simulink model "SDV_HIL"  (R2025a)
settings: Solver=VariableStepAuto  StartTime=0.0  StopTime=9999  FixedStep=0.001  RelTol=1e-3
undefined symbols (not defined in the file): Breakpoints_Fz, Cij, dspblkCoreblockFVToolHelper, eta, Fx_total_max, g, gcbh, Iz, lambda, lf, lr, mu, phi, R_eff, Tmax, xi
libraries: simulink_extras x30, slrealtimeiplib x17, slpidlib x16, simulink x10, SignalEditorBlockLib x6, dspstat3 x5, Solver_SF x3, sl3dlib x3
(part 3 of 5)

== system SDV_HIL/Draft1/Subsystem1/Motor1/Subsystem ==
  In1 : Inport
  Add : Sum
  PID Controller : slpidlib/PID Controller  Controller=PID  Form=Parallel  TimeDomain=Continuous-time  UseExternalTs=off  SampleTime=0.001  IntegratorMethod=Forward Euler  FilterMethod=Forward Euler  ControllerParametersSource=internal  P=0  I=3.5024667128  UseKiTs=off  D=0  UseExternalDerivativeSource=off  N=100  UseFilter=on  TunerSelectOption=Transfer Function Based (PID Tuner App)  InitialConditionSource=internal  InitialConditionForIntegrator=0  InitialConditionForFilter=0  DifferentiatorICPrevScaledInput=0  ExternalReset=none  TrackingMode=off  Kt=1  LimitOutput=off  SatLimitsSource=internal  UpperSaturationLimit=inf  LowerSaturationLimit=-inf  LinearizeAsGain=on  AntiWindupMode=none  Kb=1  LimitIntegrator=off  UpperIntegratorSaturationLimit=inf  LowerIntegratorSaturationLimit=-inf  POutMin=[]  POutMax=[]  IOutMin=[]  IOutMax=[]  DOutMin=[]  DOutMax=[]  NOutMin=[]  NOutMax=[]  SumOutMin=[]  SumOutMax=[]  SaturationOutMin=[]  SaturationOutMax=[]  PParamMin=[]  PParamMax=[]  IParamMin=[]  IParamMax=[]  DParamMin=[]  DParamMax=[]  NParamMin=[]  NParamMax=[]  KbParamMin=[]  KbParamMax=[]  KtParamMin=[]  KtParamMax=[]  KbOutMin=[]  KbOutMax=[]  KtOutMin=[]  KtOutMax=[]  IntegratorOutMin=[]  IntegratorOutMax=[]  FilterOutMin=[]  FilterOutMax=[]  SumI1OutMin=[]  SumI1OutMax=[]  SumI2OutMin=[]  SumI2OutMax=[]  SumI3OutMin=[]  SumI3OutMax=[]  SumI4OutMin=[]  SumI4OutMax=[]  SumDOutMin=[]  SumDOutMax=[]  DifferentiatorOutMin=[]  DifferentiatorOutMax=[]  FilterDiffOutCoefMin=[]  FilterDiffOutCoefMax=[]  ReciprocalOutMin=[]  ReciprocalOutMax=[]  SumDenOutMin=[]  SumDenOutMax=[]  SumNumOutMin=[]  SumNumOutMax=[]  DivideOutMin=[]  DivideOutMax=[]  UdiffTsProdOutMin=[]  UdiffTsProdOutMax=[]  NTsProdOutMin=[]  NTsProdOutMax=[]  UintegralTsProdOutMin=[]  UintegralTsProdOutMax=[]  UngainTsProdOutMin=[]  UngainTsProdOutMax=[]  ClampingZeroOutDataTypeStr=Inherit: Inherit via back propagation  ClampingZeroOutMin=[]  ClampingZeroOutMax=[]  FilterDenConstantOutDataTypeStr=Inherit: Inherit via back propagation  FilterDenConstantOutMin=[]  FilterDenConstantOutMax=[]  PCopyOutDataTypeStr=Inherit: Inherit via back propagation  PCopyOutMin=[]  PCopyOutMax=[]  NCopyOutDataTypeStr=Inherit: Inherit via back propagation  NCopyOutMin=[]  NCopyOutMax=[]  IntegratorContinuousStateAttributes=''  IntegratorStateMustResolveToSignalObject=off  IntegratorRTWStateStorageClass=Auto  FilterContinuousStateAttributes=''  FilterStateMustResolveToSignalObject=off  FilterRTWStateStorageClass=Auto  ParallelPVariant=InternalParameters  IdealPVariant=Disabled  IVariant=InternalParameters  DVariant=InternalParameters  IntegratorVariant=Continuous  SatVariant=Disabled  AWVariant=Passthrough  PCopyVariant=Disabled  TRVariant=Disabled  FdbkBlocksVariant=Forward  IdealPFdbkVariant=Disabled  SatFdbkVariant=Disabled  DerivativeFilterVariant=ContFilter  NVariant=InternalParameters  NCopyVariant=Disabled  FilterICVariant=InternalICsFilter  IntegratorICVariant=InternalICs  ExternalResetVariant=Disabled  TRSumVariant=Passthrough  SumFdbkVariant=Disabled  SumVariant=Sum_PID  TsampFilterVariant=InternalTs  TsampNgainVariant=Passthrough  TsampIntegralVariant=Disabled_SignalSpec  ExternalSaturationOutDataTypeStr=Inherit: Same as second input  DerivativeSourceVariant=ErrorSignal  PreIntVariant=InternalPreInt
  Saturation : Saturate  UpperLimit=110  LowerLimit=-110
  Scope : Scope
      settings: ActiveDisplayYMinimum=-13.749999999999996  ActiveDisplayYMaximum=123.75  DataLoggingVariableName=ScopeData10
  Scope1 : Scope  NumInputPorts=2
      settings: ActiveDisplayYMinimum=-21.066394763656298  ActiveDisplayYMaximum=122.34078579666662  DataLoggingVariableName=ScopeData13
  Scope2 : Scope
      settings: ActiveDisplayYMinimum=-17.082157059379561  ActiveDisplayYMaximum=107.74564424656792  DataLoggingVariableName=ScopeData16
  Sum : Sum  Inputs=|+-
  Temporary DC Motor model3 : TransferFcn  Numerator=[-146.29,3022.7]  Denominator=[1,117.06,3078.7]
  Out1 : Outport
  wires:
  [initialCondition] -> Add/2
  Add/1 -> Out1/1, Sum/2, Scope1/2, Scope2/1
  Temporary DC Motor model3/1 -> Add/1
  Saturation/1 -> Temporary DC Motor model3/1, Scope/1
  In1/1 -> Sum/1, Scope1/1
  Sum/1 -> PID Controller/1
  PID Controller/1 -> Saturation/1

== system SDV_HIL/Draft1/Subsystem1/Motor1/Subsystem1 ==
  In1 : Inport
  Add : Sum
  PID Controller : slpidlib/PID Controller  Controller=PID  Form=Parallel  TimeDomain=Continuous-time  UseExternalTs=off  SampleTime=0.001  IntegratorMethod=Forward Euler  FilterMethod=Forward Euler  ControllerParametersSource=internal  P=0  I=3.5024667128  UseKiTs=off  D=0  UseExternalDerivativeSource=off  N=100  UseFilter=on  TunerSelectOption=Transfer Function Based (PID Tuner App)  InitialConditionSource=internal  InitialConditionForIntegrator=0  InitialConditionForFilter=0  DifferentiatorICPrevScaledInput=0  ExternalReset=none  TrackingMode=off  Kt=1  LimitOutput=off  SatLimitsSource=internal  UpperSaturationLimit=inf  LowerSaturationLimit=-inf  LinearizeAsGain=on  AntiWindupMode=none  Kb=1  LimitIntegrator=off  UpperIntegratorSaturationLimit=inf  LowerIntegratorSaturationLimit=-inf  POutMin=[]  POutMax=[]  IOutMin=[]  IOutMax=[]  DOutMin=[]  DOutMax=[]  NOutMin=[]  NOutMax=[]  SumOutMin=[]  SumOutMax=[]  SaturationOutMin=[]  SaturationOutMax=[]  PParamMin=[]  PParamMax=[]  IParamMin=[]  IParamMax=[]  DParamMin=[]  DParamMax=[]  NParamMin=[]  NParamMax=[]  KbParamMin=[]  KbParamMax=[]  KtParamMin=[]  KtParamMax=[]  KbOutMin=[]  KbOutMax=[]  KtOutMin=[]  KtOutMax=[]  IntegratorOutMin=[]  IntegratorOutMax=[]  FilterOutMin=[]  FilterOutMax=[]  SumI1OutMin=[]  SumI1OutMax=[]  SumI2OutMin=[]  SumI2OutMax=[]  SumI3OutMin=[]  SumI3OutMax=[]  SumI4OutMin=[]  SumI4OutMax=[]  SumDOutMin=[]  SumDOutMax=[]  DifferentiatorOutMin=[]  DifferentiatorOutMax=[]  FilterDiffOutCoefMin=[]  FilterDiffOutCoefMax=[]  ReciprocalOutMin=[]  ReciprocalOutMax=[]  SumDenOutMin=[]  SumDenOutMax=[]  SumNumOutMin=[]  SumNumOutMax=[]  DivideOutMin=[]  DivideOutMax=[]  UdiffTsProdOutMin=[]  UdiffTsProdOutMax=[]  NTsProdOutMin=[]  NTsProdOutMax=[]  UintegralTsProdOutMin=[]  UintegralTsProdOutMax=[]  UngainTsProdOutMin=[]  UngainTsProdOutMax=[]  ClampingZeroOutDataTypeStr=Inherit: Inherit via back propagation  ClampingZeroOutMin=[]  ClampingZeroOutMax=[]  FilterDenConstantOutDataTypeStr=Inherit: Inherit via back propagation  FilterDenConstantOutMin=[]  FilterDenConstantOutMax=[]  PCopyOutDataTypeStr=Inherit: Inherit via back propagation  PCopyOutMin=[]  PCopyOutMax=[]  NCopyOutDataTypeStr=Inherit: Inherit via back propagation  NCopyOutMin=[]  NCopyOutMax=[]  IntegratorContinuousStateAttributes=''  IntegratorStateMustResolveToSignalObject=off  IntegratorRTWStateStorageClass=Auto  FilterContinuousStateAttributes=''  FilterStateMustResolveToSignalObject=off  FilterRTWStateStorageClass=Auto  ParallelPVariant=InternalParameters  IdealPVariant=Disabled  IVariant=InternalParameters  DVariant=InternalParameters  IntegratorVariant=Continuous  SatVariant=Disabled  AWVariant=Passthrough  PCopyVariant=Disabled  TRVariant=Disabled  FdbkBlocksVariant=Forward  IdealPFdbkVariant=Disabled  SatFdbkVariant=Disabled  DerivativeFilterVariant=ContFilter  NVariant=InternalParameters  NCopyVariant=Disabled  FilterICVariant=InternalICsFilter  IntegratorICVariant=InternalICs  ExternalResetVariant=Disabled  TRSumVariant=Passthrough  SumFdbkVariant=Disabled  SumVariant=Sum_PID  TsampFilterVariant=InternalTs  TsampNgainVariant=Passthrough  TsampIntegralVariant=Disabled_SignalSpec  ExternalSaturationOutDataTypeStr=Inherit: Same as second input  DerivativeSourceVariant=ErrorSignal  PreIntVariant=InternalPreInt
  Saturation : Saturate  UpperLimit=110  LowerLimit=-110
  Scope : Scope
      settings: ActiveDisplayYMinimum=-1  ActiveDisplayYMaximum=1  DataLoggingVariableName=ScopeData10
  Scope1 : Scope  NumInputPorts=2
      settings: ActiveDisplayYMinimum=70.760540850772571  ActiveDisplayYMaximum=162.62283553098897  DataLoggingVariableName=ScopeData13
  Scope2 : Scope
      settings: ActiveDisplayYMinimum=-1  ActiveDisplayYMaximum=1  DataLoggingVariableName=ScopeData16
  Sum : Sum  Inputs=|+-
  Temporary DC Motor model3 : TransferFcn  Numerator=[-146.29,3022.7]  Denominator=[1,117.06,3078.7]
  Out1 : Outport
  wires:
  PID Controller/1 -> Saturation/1
  Sum/1 -> PID Controller/1
  In1/1 -> Scope1/1, Sum/1
  Saturation/1 -> Scope/1, Temporary DC Motor model3/1
  Temporary DC Motor model3/1 -> Add/1
  Add/1 -> Scope2/1, Scope1/2, Sum/2, Out1/1
  [initialCondition] -> Add/2

== system SDV_HIL/Draft1/Subsystem1/Motor1/Subsystem2 ==
  In1 : Inport
  Add : Sum
  PID Controller : slpidlib/PID Controller  Controller=PID  Form=Parallel  TimeDomain=Continuous-time  UseExternalTs=off  SampleTime=0.001  IntegratorMethod=Forward Euler  FilterMethod=Forward Euler  ControllerParametersSource=internal  P=0  I=3.5024667128  UseKiTs=off  D=0  UseExternalDerivativeSource=off  N=100  UseFilter=on  TunerSelectOption=Transfer Function Based (PID Tuner App)  InitialConditionSource=internal  InitialConditionForIntegrator=0  InitialConditionForFilter=0  DifferentiatorICPrevScaledInput=0  ExternalReset=none  TrackingMode=off  Kt=1  LimitOutput=off  SatLimitsSource=internal  UpperSaturationLimit=inf  LowerSaturationLimit=-inf  LinearizeAsGain=on  AntiWindupMode=none  Kb=1  LimitIntegrator=off  UpperIntegratorSaturationLimit=inf  LowerIntegratorSaturationLimit=-inf  POutMin=[]  POutMax=[]  IOutMin=[]  IOutMax=[]  DOutMin=[]  DOutMax=[]  NOutMin=[]  NOutMax=[]  SumOutMin=[]  SumOutMax=[]  SaturationOutMin=[]  SaturationOutMax=[]  PParamMin=[]  PParamMax=[]  IParamMin=[]  IParamMax=[]  DParamMin=[]  DParamMax=[]  NParamMin=[]  NParamMax=[]  KbParamMin=[]  KbParamMax=[]  KtParamMin=[]  KtParamMax=[]  KbOutMin=[]  KbOutMax=[]  KtOutMin=[]  KtOutMax=[]  IntegratorOutMin=[]  IntegratorOutMax=[]  FilterOutMin=[]  FilterOutMax=[]  SumI1OutMin=[]  SumI1OutMax=[]  SumI2OutMin=[]  SumI2OutMax=[]  SumI3OutMin=[]  SumI3OutMax=[]  SumI4OutMin=[]  SumI4OutMax=[]  SumDOutMin=[]  SumDOutMax=[]  DifferentiatorOutMin=[]  DifferentiatorOutMax=[]  FilterDiffOutCoefMin=[]  FilterDiffOutCoefMax=[]  ReciprocalOutMin=[]  ReciprocalOutMax=[]  SumDenOutMin=[]  SumDenOutMax=[]  SumNumOutMin=[]  SumNumOutMax=[]  DivideOutMin=[]  DivideOutMax=[]  UdiffTsProdOutMin=[]  UdiffTsProdOutMax=[]  NTsProdOutMin=[]  NTsProdOutMax=[]  UintegralTsProdOutMin=[]  UintegralTsProdOutMax=[]  UngainTsProdOutMin=[]  UngainTsProdOutMax=[]  ClampingZeroOutDataTypeStr=Inherit: Inherit via back propagation  ClampingZeroOutMin=[]  ClampingZeroOutMax=[]  FilterDenConstantOutDataTypeStr=Inherit: Inherit via back propagation  FilterDenConstantOutMin=[]  FilterDenConstantOutMax=[]  PCopyOutDataTypeStr=Inherit: Inherit via back propagation  PCopyOutMin=[]  PCopyOutMax=[]  NCopyOutDataTypeStr=Inherit: Inherit via back propagation  NCopyOutMin=[]  NCopyOutMax=[]  IntegratorContinuousStateAttributes=''  IntegratorStateMustResolveToSignalObject=off  IntegratorRTWStateStorageClass=Auto  FilterContinuousStateAttributes=''  FilterStateMustResolveToSignalObject=off  FilterRTWStateStorageClass=Auto  ParallelPVariant=InternalParameters  IdealPVariant=Disabled  IVariant=InternalParameters  DVariant=InternalParameters  IntegratorVariant=Continuous  SatVariant=Disabled  AWVariant=Passthrough  PCopyVariant=Disabled  TRVariant=Disabled  FdbkBlocksVariant=Forward  IdealPFdbkVariant=Disabled  SatFdbkVariant=Disabled  DerivativeFilterVariant=ContFilter  NVariant=InternalParameters  NCopyVariant=Disabled  FilterICVariant=InternalICsFilter  IntegratorICVariant=InternalICs  ExternalResetVariant=Disabled  TRSumVariant=Passthrough  SumFdbkVariant=Disabled  SumVariant=Sum_PID  TsampFilterVariant=InternalTs  TsampNgainVariant=Passthrough  TsampIntegralVariant=Disabled_SignalSpec  ExternalSaturationOutDataTypeStr=Inherit: Same as second input  DerivativeSourceVariant=ErrorSignal  PreIntVariant=InternalPreInt
  Saturation : Saturate  UpperLimit=110  LowerLimit=-110
  Scope : Scope
      settings: ActiveDisplayYMinimum=-1  ActiveDisplayYMaximum=1  DataLoggingVariableName=ScopeData10
  Scope1 : Scope  NumInputPorts=2
      settings: ActiveDisplayYMinimum=70.760540850772571  ActiveDisplayYMaximum=162.62283553098897  DataLoggingVariableName=ScopeData13
  Scope2 : Scope
      settings: ActiveDisplayYMinimum=-1  ActiveDisplayYMaximum=1  DataLoggingVariableName=ScopeData16
  Sum : Sum  Inputs=|+-
  Temporary DC Motor model3 : TransferFcn  Numerator=[-146.29,3022.7]  Denominator=[1,117.06,3078.7]
  Out1 : Outport
  wires:
  [initialCondition] -> Add/2
  Add/1 -> Out1/1, Sum/2, Scope1/2, Scope2/1
  Temporary DC Motor model3/1 -> Add/1
  Saturation/1 -> Temporary DC Motor model3/1, Scope/1
  In1/1 -> Sum/1, Scope1/1
  Sum/1 -> PID Controller/1
  PID Controller/1 -> Saturation/1

== system SDV_HIL/Draft1/Subsystem1/Motor1/Subsystem3 ==
  In1 : Inport
  Add : Sum
  PID Controller : slpidlib/PID Controller  Controller=PID  Form=Parallel  TimeDomain=Continuous-time  UseExternalTs=off  SampleTime=0.001  IntegratorMethod=Forward Euler  FilterMethod=Forward Euler  ControllerParametersSource=internal  P=0  I=3.5024667128  UseKiTs=off  D=0  UseExternalDerivativeSource=off  N=100  UseFilter=on  TunerSelectOption=Transfer Function Based (PID Tuner App)  InitialConditionSource=internal  InitialConditionForIntegrator=0  InitialConditionForFilter=0  DifferentiatorICPrevScaledInput=0  ExternalReset=none  TrackingMode=off  Kt=1  LimitOutput=off  SatLimitsSource=internal  UpperSaturationLimit=inf  LowerSaturationLimit=-inf  LinearizeAsGain=on  AntiWindupMode=none  Kb=1  LimitIntegrator=off  UpperIntegratorSaturationLimit=inf  LowerIntegratorSaturationLimit=-inf  POutMin=[]  POutMax=[]  IOutMin=[]  IOutMax=[]  DOutMin=[]  DOutMax=[]  NOutMin=[]  NOutMax=[]  SumOutMin=[]  SumOutMax=[]  SaturationOutMin=[]  SaturationOutMax=[]  PParamMin=[]  PParamMax=[]  IParamMin=[]  IParamMax=[]  DParamMin=[]  DParamMax=[]  NParamMin=[]  NParamMax=[]  KbParamMin=[]  KbParamMax=[]  KtParamMin=[]  KtParamMax=[]  KbOutMin=[]  KbOutMax=[]  KtOutMin=[]  KtOutMax=[]  IntegratorOutMin=[]  IntegratorOutMax=[]  FilterOutMin=[]  FilterOutMax=[]  SumI1OutMin=[]  SumI1OutMax=[]  SumI2OutMin=[]  SumI2OutMax=[]  SumI3OutMin=[]  SumI3OutMax=[]  SumI4OutMin=[]  SumI4OutMax=[]  SumDOutMin=[]  SumDOutMax=[]  DifferentiatorOutMin=[]  DifferentiatorOutMax=[]  FilterDiffOutCoefMin=[]  FilterDiffOutCoefMax=[]  ReciprocalOutMin=[]  ReciprocalOutMax=[]  SumDenOutMin=[]  SumDenOutMax=[]  SumNumOutMin=[]  SumNumOutMax=[]  DivideOutMin=[]  DivideOutMax=[]  UdiffTsProdOutMin=[]  UdiffTsProdOutMax=[]  NTsProdOutMin=[]  NTsProdOutMax=[]  UintegralTsProdOutMin=[]  UintegralTsProdOutMax=[]  UngainTsProdOutMin=[]  UngainTsProdOutMax=[]  ClampingZeroOutDataTypeStr=Inherit: Inherit via back propagation  ClampingZeroOutMin=[]  ClampingZeroOutMax=[]  FilterDenConstantOutDataTypeStr=Inherit: Inherit via back propagation  FilterDenConstantOutMin=[]  FilterDenConstantOutMax=[]  PCopyOutDataTypeStr=Inherit: Inherit via back propagation  PCopyOutMin=[]  PCopyOutMax=[]  NCopyOutDataTypeStr=Inherit: Inherit via back propagation  NCopyOutMin=[]  NCopyOutMax=[]  IntegratorContinuousStateAttributes=''  IntegratorStateMustResolveToSignalObject=off  IntegratorRTWStateStorageClass=Auto  FilterContinuousStateAttributes=''  FilterStateMustResolveToSignalObject=off  FilterRTWStateStorageClass=Auto  ParallelPVariant=InternalParameters  IdealPVariant=Disabled  IVariant=InternalParameters  DVariant=InternalParameters  IntegratorVariant=Continuous  SatVariant=Disabled  AWVariant=Passthrough  PCopyVariant=Disabled  TRVariant=Disabled  FdbkBlocksVariant=Forward  IdealPFdbkVariant=Disabled  SatFdbkVariant=Disabled  DerivativeFilterVariant=ContFilter  NVariant=InternalParameters  NCopyVariant=Disabled  FilterICVariant=InternalICsFilter  IntegratorICVariant=InternalICs  ExternalResetVariant=Disabled  TRSumVariant=Passthrough  SumFdbkVariant=Disabled  SumVariant=Sum_PID  TsampFilterVariant=InternalTs  TsampNgainVariant=Passthrough  TsampIntegralVariant=Disabled_SignalSpec  ExternalSaturationOutDataTypeStr=Inherit: Same as second input  DerivativeSourceVariant=ErrorSignal  PreIntVariant=InternalPreInt
  Saturation : Saturate  UpperLimit=110  LowerLimit=-110
  Scope : Scope
      settings: ActiveDisplayYMinimum=-1  ActiveDisplayYMaximum=1  DataLoggingVariableName=ScopeData10
  Scope1 : Scope  NumInputPorts=2
      settings: ActiveDisplayYMinimum=70.760540850772571  ActiveDisplayYMaximum=162.62283553098897  DataLoggingVariableName=ScopeData13
  Scope2 : Scope
      settings: ActiveDisplayYMinimum=-1  ActiveDisplayYMaximum=1  DataLoggingVariableName=ScopeData16
  Sum : Sum  Inputs=|+-
  Temporary DC Motor model3 : TransferFcn  Numerator=[-146.29,3022.7]  Denominator=[1,117.06,3078.7]
  Out1 : Outport
  wires:
  PID Controller/1 -> Saturation/1
  Sum/1 -> PID Controller/1
  In1/1 -> Scope1/1, Sum/1
  Saturation/1 -> Scope/1, Temporary DC Motor model3/1
  Temporary DC Motor model3/1 -> Add/1
  Add/1 -> Scope2/1, Scope1/2, Sum/2, Out1/1
  [initialCondition] -> Add/2

== system SDV_HIL/Draft1/Subsystem1/Motor1/Traction Control ==
  SpdTCS : Inport
  Add : Sum
  Add1 : Sum
  Mux : Mux  Inputs=2
  Scope1 : Scope
      settings: ActiveDisplayYMinimum=-42.212003619613114  ActiveDisplayYMaximum=156.59295699794211  DataLoggingVariableName=ScopeData29
  Selector : Selector  InputPortWidth=4  IndexOptions=Index vector (dialog)  Indices=[1 2]  OutputSizes=1
  Selector1 : Selector  InputPortWidth=4  IndexOptions=Index vector (dialog)  Indices=[3 4]  OutputSizes=1
  Slip Calculation : Subsystem
  Slip Calculation1 : Subsystem
  Subsystem : Subsystem
  Subsystem1 : Subsystem
  Out1 : Outport
  wires:
  Subsystem1/1(y) -> Add1/2
  Slip Calculation1/1(slip) -> Subsystem1/1(slip)
  Slip Calculation/1(slip) -> Subsystem/1(In1)
  Subsystem/1(y) -> Add/2
  Add/1 -> Mux/1
  Add1/1 -> Mux/2
  Mux/1 -> Out1/1, Scope1/1
  Selector1/1 -> Add1/1
  Selector/1 -> Add/1
  SpdTCS/1 -> Selector1/1, Selector/1

== system SDV_HIL/Draft1/Subsystem1/Steering1/Cr, calculation ==
  In1 : Inport
  Add : Sum
  Add1 : Sum
  Demux : Demux  Outputs=2
  Divide : Product  Inputs=*/
  Divide1 : Product  Inputs=*/
  Divide2 : Product  Inputs=*/
  Scope1 : Scope
      settings: ActiveDisplayYMinimum=-33.245119024843021  ActiveDisplayYMaximum=11.158574802269591  DataLoggingVariableName=ScopeData36
  Scope2 : Scope  NumInputPorts=3
      settings: ActiveDisplayYMinimum=-11896.025438814215  ActiveDisplayYMaximum=9098.0677384906721  DataLoggingVariableName=ScopeData37
  Scope3 : Scope  NumInputPorts=2
      settings: ActiveDisplayYMinimum=-1372.0128718321157  ActiveDisplayYMaximum=6027.9532460136825  DataLoggingVariableName=ScopeData39
  Scope4 : Scope
      settings: ActiveDisplayYMinimum=-1233.3601043062406  ActiveDisplayYMaximum=4986.210757668915  DataLoggingVariableName=ScopeData46
  Scope5 : Scope
      settings: ActiveDisplayYMinimum=-54160.327682168427  ActiveDisplayYMaximum=53171.641125613256  DataLoggingVariableName=ScopeData12
  Selector : Selector  InputPortWidth=4  IndexOptions=Index vector (dialog)  Indices=[3 4]  OutputSizes=1
  Subsystem : Subsystem
  wires:
  Add1/1 -> Scope5/1  "Cr"
  [sideslip_R2] -> Divide2/2
  Divide2/1 -> Add1/2  "Cr_R2"
  Divide1/1 -> Add1/1  "Cr_L2"
  [sideslip_L2] -> Divide1/2
  Divide/1 -> Scope2/2  "Cr"
  Add/1 -> Divide/1, Scope2/1, Scope3/2
  Selector/1 -> Demux/1, Scope3/1
  Demux/2 -> Add/2, Divide2/1
  Subsystem/1(Out1) -> Scope1/1, Scope2/3, Divide/2  "ar, side slip rear"
  [Fy] -> Selector/1, Scope4/1
  Demux/1 -> Divide1/1, Add/1
  In1/1 -> Subsystem/1(In1)

== system SDV_HIL/Draft1/Subsystem1/Steering1/Dynamic ==
  In2 : Inport
  Mz : Inport  Port=2
  Demux : Demux
  Mux : Mux
  PID Controller{,1..3} (4 alike) : slpidlib/PID Controller  Controller=PD  Form=Parallel  TimeDomain=Continuous-time  UseExternalTs=off  SampleTime=-1  IntegratorMethod=Forward Euler  FilterMethod=Forward Euler  ControllerParametersSource=internal  P=447.054647999311  I=1.94153008706553  UseKiTs=off  D=0  UseExternalDerivativeSource=off  N=100  UseFilter=on  TunerSelectOption=Transfer Function Based (PID Tuner App)  InitialConditionSource=internal  InitialConditionForIntegrator=0  InitialConditionForFilter=0  DifferentiatorICPrevScaledInput=0  ExternalReset=none  TrackingMode=off  Kt=1  LimitOutput=off  SatLimitsSource=internal  UpperSaturationLimit=inf  LowerSaturationLimit=-inf  LinearizeAsGain=on  AntiWindupMode=none  Kb=1  LimitIntegrator=off  UpperIntegratorSaturationLimit=inf  LowerIntegratorSaturationLimit=-inf  POutMin=[]  POutMax=[]  IOutMin=[]  IOutMax=[]  DOutMin=[]  DOutMax=[]  NOutMin=[]  NOutMax=[]  SumOutMin=[]  SumOutMax=[]  SaturationOutMin=[]  SaturationOutMax=[]  PParamMin=[]  PParamMax=[]  IParamMin=[]  IParamMax=[]  DParamMin=[]  DParamMax=[]  NParamMin=[]  NParamMax=[]  KbParamMin=[]  KbParamMax=[]  KtParamMin=[]  KtParamMax=[]  KbOutMin=[]  KbOutMax=[]  KtOutMin=[]  KtOutMax=[]  IntegratorOutMin=[]  IntegratorOutMax=[]  FilterOutMin=[]  FilterOutMax=[]  SumI1OutMin=[]  SumI1OutMax=[]  SumI2OutMin=[]  SumI2OutMax=[]  SumI3OutMin=[]  SumI3OutMax=[]  SumI4OutMin=[]  SumI4OutMax=[]  SumDOutMin=[]  SumDOutMax=[]  DifferentiatorOutMin=[]  DifferentiatorOutMax=[]  FilterDiffOutCoefMin=[]  FilterDiffOutCoefMax=[]  ReciprocalOutMin=[]  ReciprocalOutMax=[]  SumDenOutMin=[]  SumDenOutMax=[]  SumNumOutMin=[]  SumNumOutMax=[]  DivideOutMin=[]  DivideOutMax=[]  UdiffTsProdOutMin=[]  UdiffTsProdOutMax=[]  NTsProdOutMin=[]  NTsProdOutMax=[]  UintegralTsProdOutMin=[]  UintegralTsProdOutMax=[]  UngainTsProdOutMin=[]  UngainTsProdOutMax=[]  ClampingZeroOutDataTypeStr=Inherit: Inherit via back propagation  ClampingZeroOutMin=[]  ClampingZeroOutMax=[]  FilterDenConstantOutDataTypeStr=Inherit: Inherit via back propagation  FilterDenConstantOutMin=[]  FilterDenConstantOutMax=[]  PCopyOutDataTypeStr=Inherit: Inherit via back propagation  PCopyOutMin=[]  PCopyOutMax=[]  NCopyOutDataTypeStr=Inherit: Inherit via back propagation  NCopyOutMin=[]  NCopyOutMax=[]  IntegratorContinuousStateAttributes=''  IntegratorStateMustResolveToSignalObject=off  IntegratorRTWStateStorageClass=Auto  FilterContinuousStateAttributes=''  FilterStateMustResolveToSignalObject=off  FilterRTWStateStorageClass=Auto  ParallelPVariant=InternalParameters  IdealPVariant=Disabled  IVariant=Disabled  DVariant=InternalParameters  IntegratorVariant=Disabled  SatVariant=Disabled  AWVariant=Disabled  PCopyVariant=Disabled  TRVariant=Disabled  FdbkBlocksVariant=Forward  IdealPFdbkVariant=Disabled  SatFdbkVariant=Disabled  DerivativeFilterVariant=ContFilter  NVariant=InternalParameters  NCopyVariant=Disabled  FilterICVariant=InternalICsFilter  IntegratorICVariant=Disabled  ExternalResetVariant=Disabled  TRSumVariant=Passthrough  SumFdbkVariant=Disabled  SumVariant=Sum_PD  TsampFilterVariant=InternalTs  TsampNgainVariant=Passthrough  TsampIntegralVariant=Disabled_SignalSpec  ExternalSaturationOutDataTypeStr=Inherit: Same as second input  DerivativeSourceVariant=ErrorSignal  PreIntVariant=InternalPreInt
  Scope{,1..3} (4 alike) : Scope  NumInputPorts=2
      Scope settings: ActiveDisplayYMinimum=-1  ActiveDisplayYMaximum=1
      Scope1 settings: ActiveDisplayYMinimum=1.8720993876921048  ActiveDisplayYMaximum=2.8130930610708664  DataLoggingVariableName=ScopeData32
      Scope2 settings: ActiveDisplayYMinimum=-18267.79992914902  ActiveDisplayYMaximum=55993.76279968489  DataLoggingVariableName=ScopeData58
      Scope3 settings: ActiveDisplayYMinimum=-0.014012303296182898  ActiveDisplayYMaximum=0.010807485381998104  DataLoggingVariableName=ScopeData59
  Steering cmd : Subsystem
  Sum{,1..5} (6 alike) : Sum  Inputs=|+-
  Temporary Stepper Motor model{1..4} (4 alike) : TransferFcn  Numerator=[80.823,1752.8]  Denominator=[1,177.23,1759.6]
  Deg : Outport
  wires:
  Sum2/1 -> Scope3/1, PID Controller2/1
  Sum3/1 -> PID Controller3/1, Scope3/2
  Steering cmd/1(Out1) -> Sum5/2, Sum4/2
  Sum5/1 -> Scope/2, Sum3/1
  Demux/4 -> Sum5/1
  Sum4/1 -> Scope/1, Sum2/1
  Demux/3 -> Sum4/1
  Mz/1 -> Steering cmd/1(In1)
  Demux/2 -> Sum1/1
  Sum1/1 -> PID Controller1/1
  Demux/1 -> Sum/1
  Sum/1 -> PID Controller/1
  PID Controller3/1 -> Temporary Stepper Motor model4/1, Scope2/2
  PID Controller2/1 -> Temporary Stepper Motor model3/1, Scope2/1
  PID Controller1/1 -> Temporary Stepper Motor model2/1
  PID Controller/1 -> Temporary Stepper Motor model1/1
  Mux/1 -> Deg/1
  Temporary Stepper Motor model4/1 -> Mux/4, Scope1/1, Sum3/2
  Temporary Stepper Motor model3/1 -> Mux/3, Scope1/2, Sum2/2
  Temporary Stepper Motor model2/1 -> Mux/2, Sum1/2
  Temporary Stepper Motor model1/1 -> Mux/1, Sum/2
  In2/1 -> Demux/1

== system SDV_HIL/Draft1/UDP Transmit PC -> VCU1/Subsystem/4 Wheel Steering system ==
  Spd : Inport
  Str : Inport  Port=2
  Display : Display
  Display1 : Display
  Kinematik : Subsystem
  Ang_reff : Outport
  wires:
  Kinematik/2(YO) -> Display/1
  Kinematik/3(XO) -> Display1/1
  Str/1 -> Kinematik/2(Steer)
  Spd/1 -> Kinematik/1(Speed)
  Kinematik/1(Out1) -> Ang_reff/1

== system SDV_HIL/Draft1/UDP Transmit PC -> VCU1/Subsystem/Torque Vectoring ==
  Vx_des : Inport
  Vx : Inport  Port=2
  Vy : Inport  Port=3
  AngWheel : Inport  Port=4
  r : Inport  Port=5
  Fy : Inport  Port=6
  Fz : Inport  Port=7  PortDimensions=[4 1]
  Ca Calculations : Subsystem
  Constant : Constant  Value=0
  Lower-Level Control : Subsystem
      settings: PortSchema="{\"entries\":[{\"content\":{\"sides\":[{\"content\":{\"connectorIds\":[\"In1\",\"In2\"]},\"type\":\"ConnectorPlacement.EquallySpacedRectSide\",\"uuid\":\"57e37133-a4ce-4bcd-b7d5-2c7ad964fba5\"},{\"content\":{\"connectorIds\":[\"Out1\"],\"side\":\"RIGHT\"},\"type\":\"ConnectorPlacement.EquallySpacedRectSide\",\"uuid\":\"b1a2d58e-03dd-4a8c-b0ff-f0fba1e94d60\"},{\"content\":{\"side\":\"TOP\"},\"type\":\"ConnectorPlacement.EquallySpacedRectSide\",\"uuid\":\"ceca0281-a87d-4fe2-92d9-19deb493506e\"},{\"content\":{\"connectorIds\":[\"In3\",\"In4\"],\"side\":\"BOTTOM\"},\"type\":\"ConnectorPlacement.EquallySpacedRectSide\",\"uuid\":\"a2fed640-7310-4b0a-b340-bd8e53025f92\"}]},\"type\":\"ConnectorPlacement.EquallySpacedConnector\",\"uuid\":\"a7bc2132-8edf-46cf-bd03-69d09e070427\"}],\"packageUris\":[\"http://schema.mathworks.com/mf0/Connector/R2020b\"],\"version\":\"1.0\"}"
  Reference Model : Subsystem
  Scope1 : Scope  Commented=on
      settings: TimeSpan=10  ActiveDisplayYMinimum=-27041.642916219451  ActiveDisplayYMaximum=46357.700395381871  DataLoggingVariableName=ScopeData5
  Scope2 : Scope  Commented=on
      settings: TimeSpan=10  ActiveDisplayYMinimum=-266.81339424220005  ActiveDisplayYMaximum=314.09270908605555  DataLoggingVariableName=ScopeData7
  Speed Control : Subsystem
  Terminator : Terminator
  Upper-Level Control : Subsystem
      settings: PortSchema="{\"entries\":[{\"content\":{\"sides\":[{\"content\":{\"connectorIds\":[\"In1\",\"In2\"]},\"type\":\"ConnectorPlacement.EquallySpacedRectSide\",\"uuid\":\"0439ec5c-b28f-4113-9d52-608e9559868e\"},{\"content\":{\"connectorIds\":[\"Out1\"],\"side\":\"RIGHT\"},\"type\":\"ConnectorPlacement.EquallySpacedRectSide\",\"uuid\":\"fb34909b-3fa5-4238-9bd9-6fa6bbc40fd8\"},{\"content\":{\"side\":\"TOP\"},\"type\":\"ConnectorPlacement.EquallySpacedRectSide\",\"uuid\":\"fd4c258c-89bb-45ab-b8b8-d01502b1a89c\"},{\"content\":{\"connectorIds\":[\"In3\",\"In4\",\"In5\",\"In6\"],\"side\":\"BOTTOM\"},\"type\":\"ConnectorPlacement.EquallySpacedRectSide\",\"uuid\":\"b800e5eb-1f42-45fc-807a-e4c0534ff65a\"}]},\"type\":\"ConnectorPlacement.EquallySpacedConnector\",\"uuid\":\"9af4ca01-5bc7-46a7-8cf4-646798371eaa\"}],\"packageUris\":[\"http://schema.mathworks.com/mf0/Connector/R2020b\"],\"version\":\"1.0\"}"
  beta Calculations : Subsystem
  delta_in Calculations : Subsystem
  TqMotorRef : Outport
  Mzd : Outport  Port=2
  tag scope: beta=global, r_des=global
  wires:
  Fz/1 -> Ca Calculations/1(<Fz>), Lower-Level Control/4(Fz)
  Reference Model/1(r_des) -> [r_des], Upper-Level Control/1(r_des)
  Speed Control/1(Fx_total) -> Lower-Level Control/1(Fx_total)
  beta Calculations/1(beta) -> [beta], Upper-Level Control/4(beta)
  Vx/1 -> beta Calculations/1(Vx), Speed Control/2(Vx), Reference Model/2(Vx)
  Vx_des/1 -> Speed Control/1(Vx_des)
  r/1 -> Upper-Level Control/3(r)
  Fy/1 -> Upper-Level Control/6(Fy)
  Ca Calculations/1(Ca) -> Reference Model/3(Ca)
  Lower-Level Control/1(TqMotorRef) -> TqMotorRef/1, Scope2/1  "Tqwheel"
  AngWheel/1 -> delta_in Calculations/1(AngWheel)
  delta_in Calculations/1(delta_in) -> Lower-Level Control/3(delta_in), Upper-Level Control/5(delta_in), Reference Model/1(delta_in)
  Vy/1 -> beta Calculations/2(Vy)
  Upper-Level Control/1(Mzd) -> Lower-Level Control/2(Mzd), Mzd/1, Scope1/1
  Constant/1 -> Upper-Level Control/2(beta_des)
  Reference Model/2(beta_des) -> Terminator/1

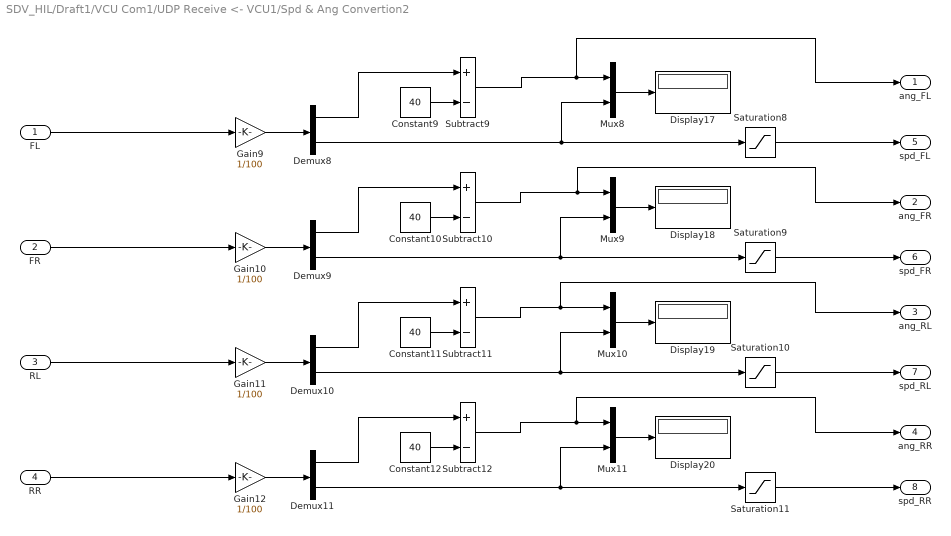
== system SDV_HIL/Draft1/VCU Com1/UDP Receive <- VCU1/Spd & Ang Convertion2 ==
  FL : Inport
  FR : Inport  Port=2
  RL : Inport  Port=3
  RR : Inport  Port=4
  Constant{9..12} (4 alike) : Constant  Value=40
  Demux{8..11} (4 alike) : Demux  Outputs=2
  Display{17..20} (4 alike) : Display
  Gain{9..12} (4 alike) : Gain  Gain=1/100
  Mux{8..11} (4 alike) : Mux  Inputs=2
  Saturation{8..11} (4 alike) : Saturate  UpperLimit=100  LowerLimit=0
  Subtract{9..12} (4 alike) : Sum  Inputs=+-
  ang_FL : Outport
  ang_FR : Outport  Port=2
  ang_RL : Outport  Port=3
  ang_RR : Outport  Port=4
  spd_FL : Outport  Port=5
  spd_FR : Outport  Port=6
  spd_RL : Outport  Port=7
  spd_RR : Outport  Port=8
  wires:
  Demux8/1 -> Subtract9/1
  Gain12/1 -> Demux11/1
  Gain9/1 -> Demux8/1
  Demux10/2 -> Mux10/2, Saturation10/1
  RR/1 -> Gain12/1
  Demux9/2 -> Saturation9/1, Mux9/2
  Demux9/1 -> Subtract10/1
  FR/1 -> Gain10/1
  Subtract11/1 -> ang_RL/1, Mux10/1
  Subtract9/1 -> ang_FL/1, Mux8/1
  Gain10/1 -> Demux9/1
  Subtract10/1 -> ang_FR/1, Mux9/1
  Constant10/1 -> Subtract10/2
  Mux9/1 -> Display18/1
  Mux8/1 -> Display17/1
  FL/1 -> Gain9/1
  Subtract12/1 -> ang_RR/1, Mux11/1
  Demux11/2 -> Mux11/2, Saturation11/1
  Mux10/1 -> Display19/1
  Saturation11/1 -> spd_RR/1
  Demux10/1 -> Subtract11/1
  Demux11/1 -> Subtract12/1
  Constant12/1 -> Subtract12/2
  Mux11/1 -> Display20/1
  Gain11/1 -> Demux10/1
  Demux8/2 -> Mux8/2, Saturation8/1
  Constant11/1 -> Subtract11/2
  Saturation8/1 -> spd_FL/1
  Constant9/1 -> Subtract9/2
  Saturation9/1 -> spd_FR/1
  RL/1 -> Gain11/1
  Saturation10/1 -> spd_RL/1

== system SDV_HIL/HIL/UDP Transmit PC -> VCU/Subsystem/4 Wheel Steering system ==
  Spd : Inport
  Str : Inport  Port=2
  Display : Display
  Display1 : Display
  Kinematik : Subsystem
  Ang_reff : Outport
  wires:
  Kinematik/2(YO) -> Display/1
  Kinematik/3(XO) -> Display1/1
  Str/1 -> Kinematik/2(Steer)
  Spd/1 -> Kinematik/1(Speed)
  Kinematik/1(Out1) -> Ang_reff/1

== system SDV_HIL/HIL/UDP Transmit PC -> VCU/Subsystem/Torque Vectoring ==
  Vx_des : Inport
  Vx : Inport  Port=2
  Vy : Inport  Port=3
  AngWheel : Inport  Port=4
  r : Inport  Port=5
  Fy : Inport  Port=6
  Fz : Inport  Port=7  PortDimensions=[4 1]
  Ca Calculations : Subsystem
  Constant : Constant  Value=0
  Lower-Level Control : Subsystem
      settings: PortSchema="{\"entries\":[{\"content\":{\"sides\":[{\"content\":{\"connectorIds\":[\"In1\",\"In2\"]},\"type\":\"ConnectorPlacement.EquallySpacedRectSide\",\"uuid\":\"57e37133-a4ce-4bcd-b7d5-2c7ad964fba5\"},{\"content\":{\"connectorIds\":[\"Out1\"],\"side\":\"RIGHT\"},\"type\":\"ConnectorPlacement.EquallySpacedRectSide\",\"uuid\":\"b1a2d58e-03dd-4a8c-b0ff-f0fba1e94d60\"},{\"content\":{\"side\":\"TOP\"},\"type\":\"ConnectorPlacement.EquallySpacedRectSide\",\"uuid\":\"ceca0281-a87d-4fe2-92d9-19deb493506e\"},{\"content\":{\"connectorIds\":[\"In3\",\"In4\"],\"side\":\"BOTTOM\"},\"type\":\"ConnectorPlacement.EquallySpacedRectSide\",\"uuid\":\"a2fed640-7310-4b0a-b340-bd8e53025f92\"}]},\"type\":\"ConnectorPlacement.EquallySpacedConnector\",\"uuid\":\"a7bc2132-8edf-46cf-bd03-69d09e070427\"}],\"packageUris\":[\"http://schema.mathworks.com/mf0/Connector/R2020b\"],\"version\":\"1.0\"}"
  Reference Model : Subsystem
  Scope1 : Scope  Commented=on
      settings: TimeSpan=10  ActiveDisplayYMinimum=-27041.642916219451  ActiveDisplayYMaximum=46357.700395381871  DataLoggingVariableName=ScopeData5
  Scope2 : Scope  Commented=on
      settings: TimeSpan=10  ActiveDisplayYMinimum=-266.81339424220005  ActiveDisplayYMaximum=314.09270908605555  DataLoggingVariableName=ScopeData7
  Speed Control : Subsystem
  Terminator : Terminator
  Upper-Level Control : Subsystem
      settings: PortSchema="{\"entries\":[{\"content\":{\"sides\":[{\"content\":{\"connectorIds\":[\"In1\",\"In2\"]},\"type\":\"ConnectorPlacement.EquallySpacedRectSide\",\"uuid\":\"0439ec5c-b28f-4113-9d52-608e9559868e\"},{\"content\":{\"connectorIds\":[\"Out1\"],\"side\":\"RIGHT\"},\"type\":\"ConnectorPlacement.EquallySpacedRectSide\",\"uuid\":\"fb34909b-3fa5-4238-9bd9-6fa6bbc40fd8\"},{\"content\":{\"side\":\"TOP\"},\"type\":\"ConnectorPlacement.EquallySpacedRectSide\",\"uuid\":\"fd4c258c-89bb-45ab-b8b8-d01502b1a89c\"},{\"content\":{\"connectorIds\":[\"In3\",\"In4\",\"In5\",\"In6\"],\"side\":\"BOTTOM\"},\"type\":\"ConnectorPlacement.EquallySpacedRectSide\",\"uuid\":\"b800e5eb-1f42-45fc-807a-e4c0534ff65a\"}]},\"type\":\"ConnectorPlacement.EquallySpacedConnector\",\"uuid\":\"9af4ca01-5bc7-46a7-8cf4-646798371eaa\"}],\"packageUris\":[\"http://schema.mathworks.com/mf0/Connector/R2020b\"],\"version\":\"1.0\"}"
  beta Calculations : Subsystem
  delta_in Calculations : Subsystem
  TqMotorRef : Outport
  Mzd : Outport  Port=2
  tag scope: beta=global, r_des=global
  wires:
  Fz/1 -> Ca Calculations/1(<Fz>), Lower-Level Control/4(Fz)
  Reference Model/1(r_des) -> [r_des], Upper-Level Control/1(r_des)
  Speed Control/1(Fx_total) -> Lower-Level Control/1(Fx_total)
  beta Calculations/1(beta) -> [beta], Upper-Level Control/4(beta)
  Vx/1 -> beta Calculations/1(Vx), Speed Control/2(Vx), Reference Model/2(Vx)
  Vx_des/1 -> Speed Control/1(Vx_des)
  r/1 -> Upper-Level Control/3(r)
  Fy/1 -> Upper-Level Control/6(Fy)
  Ca Calculations/1(Ca) -> Reference Model/3(Ca)
  Lower-Level Control/1(TqMotorRef) -> TqMotorRef/1, Scope2/1  "Tqwheel"
  AngWheel/1 -> delta_in Calculations/1(AngWheel)
  delta_in Calculations/1(delta_in) -> Lower-Level Control/3(delta_in), Upper-Level Control/5(delta_in), Reference Model/1(delta_in)
  Vy/1 -> beta Calculations/2(Vy)
  Upper-Level Control/1(Mzd) -> Lower-Level Control/2(Mzd), Mzd/1, Scope1/1
  Constant/1 -> Upper-Level Control/2(beta_des)
  Reference Model/2(beta_des) -> Terminator/1

== system SDV_HIL/Draft1/Subsystem1/Motor1/Traction Control/Slip Calculation ==
  Constant : Constant  Value=0.5
  Divide : Product  Inputs=*/
  Max : MinMax  Function=max  Inputs=2
  Mux : Mux  Inputs=2
  Subtract : Sum  Inputs=+-
  slip : Outport
  wires:
  Mux/1 -> Subtract/1
  [Vx_R1] -> Mux/2
  [Vx_L1] -> Mux/1
  Constant/1 -> Max/2
  Max/1 -> Divide/2
  [Vx] -> Subtract/2, Max/1
  Divide/1 -> slip/1  "slip"
  Subtract/1 -> Divide/1

== system SDV_HIL/Draft1/Subsystem1/Motor1/Traction Control/Slip Calculation1 ==
  Constant : Constant  Value=0.5
  Divide : Product  Inputs=*/
  Max : MinMax  Function=max  Inputs=2
  Mux : Mux  Inputs=2
  Subtract : Sum  Inputs=+-
  slip : Outport
  wires:
  Subtract/1 -> Divide/1
  Divide/1 -> slip/1  "slip"
  [Vx] -> Max/1, Subtract/2
  Max/1 -> Divide/2
  Constant/1 -> Max/2
  [Vx_L2] -> Mux/1
  [Vx_R2] -> Mux/2
  Mux/1 -> Subtract/1

== system SDV_HIL/Draft1/Subsystem1/Motor1/Traction Control/Subsystem ==
  In1 : Inport
  Add : Sum
  Constant : Constant  Value=0
  Derivative : Derivative
  Gain : Gain
  Gain1 : Gain  Gain=0.3
  Gain2 : Gain  Gain=1/0.3
  Gain3 : Gain  Gain=80
  Rate Transition : RateTransition  OutPortSampleTime=0.001
  Saturation : Saturate  UpperLimit=1  LowerLimit=-1
  Scope : Scope
      settings: ActiveDisplayYMinimum=-125  ActiveDisplayYMaximum=125  DataLoggingVariableName=ScopeData4
  Scope4 : Scope  NumInputPorts=2
      settings: ActiveDisplayYMinimum=-0.01807026937400167  ActiveDisplayYMaximum=0.025518988518367734  DataLoggingVariableName=ScopeData26
  Sum4 : Sum  Inputs=|+-
  y : Outport
  wires:
  Rate Transition/1 -> Gain/1, Gain1/1
  Saturation/1 -> Gain3/1
  Gain2/1 -> Saturation/1
  Add/1 -> Gain2/1
  Derivative/1 -> Add/2
  Gain1/1 -> Derivative/1
  Gain/1 -> Add/1
  Gain3/1 -> y/1, Scope/1
  Sum4/1 -> Rate Transition/1
  In1/1 -> Scope4/2, Sum4/2
  Constant/1 -> Sum4/1, Scope4/1

== system SDV_HIL/Draft1/Subsystem1/Motor1/Traction Control/Subsystem1 ==
  slip : Inport
  Add : Sum
  Constant : Constant  Value=0
  Derivative : Derivative
  Gain : Gain
  Gain1 : Gain  Gain=0.3
  Gain2 : Gain  Gain=1/0.3
  Gain3 : Gain  Gain=80
  Rate Transition : RateTransition  OutPortSampleTime=0.001
  Saturation : Saturate  UpperLimit=1  LowerLimit=-1
  Scope : Scope
      settings: ActiveDisplayYMinimum=-125  ActiveDisplayYMaximum=125  DataLoggingVariableName=ScopeData4
  Scope4 : Scope  NumInputPorts=2
      settings: ActiveDisplayYMinimum=-2.0907549275635615  ActiveDisplayYMaximum=6.7023982861737288  DataLoggingVariableName=ScopeData26
  Sum4 : Sum  Inputs=|+-
  y : Outport
  wires:
  Constant/1 -> Scope4/1, Sum4/1
  slip/1 -> Sum4/2, Scope4/2
  Sum4/1 -> Rate Transition/1
  Gain3/1 -> Scope/1, y/1
  Gain/1 -> Add/1
  Gain1/1 -> Derivative/1
  Derivative/1 -> Add/2
  Add/1 -> Gain2/1
  Gain2/1 -> Saturation/1
  Saturation/1 -> Gain3/1
  Rate Transition/1 -> Gain1/1, Gain/1

== system SDV_HIL/Draft1/Subsystem1/Steering1/Cr, calculation/Subsystem ==
  In1 : Inport
  Add : Sum
  Add1 : Sum
  Degrees to Radians : simulink_extras/Transformations/Degrees to Radians
  Demux : Demux  Outputs=2
  Divide : Product  Inputs=*/
  Gain : Gain  Gain=1/2
  Gain1 : Gain  Gain=2297.5
  Gain2 : Gain  Gain=1/3.6
  Gain3 : Gain  Gain=1/3.6
  Scope : Scope
      settings: ActiveDisplayYMinimum=-1  ActiveDisplayYMaximum=1  DataLoggingVariableName=ScopeData49
  Selector : Selector  InputPortWidth=4  IndexOptions=Index vector (dialog)  Indices=[3 4]  OutputSizes=1
  Sum : Sum  Inputs=|+-
  Out1 : Outport
  wires:
  Gain3/1 -> Divide/2
  Gain2/1 -> Add1/2
  Degrees to Radians/1 -> Selector/1, Scope/1
  Sum/1 -> Out1/1
  Divide/1 -> Sum/2
  [Vx] -> Gain3/1
  Add1/1 -> Divide/1
  [Vy] -> Gain2/1
  Gain1/1 -> Add1/1
  [yawrate] -> Gain1/1
  Gain/1 -> Sum/1
  Selector/1 -> Demux/1
  Demux/2 -> Add/2
  Demux/1 -> Add/1
  Add/1 -> Gain/1
  In1/1 -> Degrees to Radians/1

== system SDV_HIL/Draft1/Subsystem1/Steering1/Dynamic/Steering cmd ==
  In1 : Inport
  Constant : Constant  Value=51430
  Divide1 : Product  Inputs=*/
  Gain : Gain
  Gain1 : Gain  Gain=2297.5
  Radians to Degrees : simulink_extras/Transformations/Radians to Degrees
  Saturation : Saturate  UpperLimit=5  LowerLimit=-5
  Scope5 : Scope
      settings: ActiveDisplayYMinimum=-0.018787262592865651  ActiveDisplayYMaximum=0.0095340990159234786  DataLoggingVariableName=ScopeData51
  Out1 : Outport
  wires:
  Gain/1 -> Divide1/1
  Divide1/1 -> Radians to Degrees/1
  Gain1/1 -> Divide1/2
  In1/1 -> Gain/1
  Constant/1 -> Gain1/1
  Saturation/1 -> Scope5/1, Out1/1
  Radians to Degrees/1 -> Saturation/1

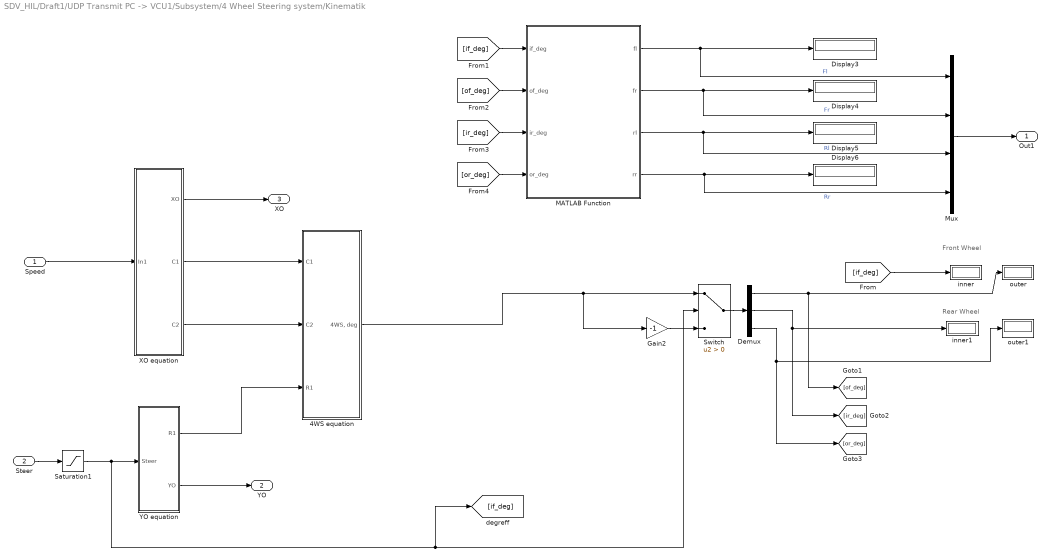
== system SDV_HIL/Draft1/UDP Transmit PC -> VCU1/Subsystem/4 Wheel Steering system/Kinematik ==
  note: Front Wheel
  note: Rear Wheel
  Speed : Inport
  Steer : Inport  Port=2
  4WS equation : Subsystem
  Demux : Demux  Outputs=3
  Display{3..6} (4 alike) : Display
  Gain2 : Gain  Gain=-1
  MATLAB Function : MATLAB Function  TreatAsAtomicUnit=on
  Mux : Mux
  Saturation1 : Saturate  UpperLimit=40  LowerLimit=-40
  Switch : Switch  Criteria=u2 > Threshold  SaturateOnIntegerOverflow=off  InputSameDT=off
  XO equation : Subsystem
  YO equation : Subsystem
  inner : Display
  inner1 : Display
  outer : Display
  outer1 : Display
  Out1 : Outport
  YO : Outport  Port=2
  XO : Outport  Port=3
  wires:
  Gain2/1 -> Switch/3
  Switch/1 -> Demux/1
  MATLAB Function/1(fl) -> Display3/1, Mux/1  "Fl"
  MATLAB Function/3(rl) -> Display5/1, Mux/3  "Rl"
  XO equation/1(XO) -> XO/1
  XO equation/2(C1) -> 4WS equation/1(C1)
  XO equation/3(C2) -> 4WS equation/2(C2)
  Steer/1 -> Saturation1/1
  YO equation/1(R1) -> 4WS equation/3(R1)
  YO equation/2(YO) -> YO/1
  4WS equation/1("4WS, deg") -> Gain2/1, Switch/1
  MATLAB Function/2(fr) -> Display4/1, Mux/2  "Fr"
  MATLAB Function/4(rr) -> Display6/1, Mux/4  "Rr"
  [if_deg] -> MATLAB Function/1(if_deg)
  [of_deg] -> MATLAB Function/2(of_deg)
  [ir_deg] -> MATLAB Function/3(ir_deg)
  [or_deg] -> MATLAB Function/4(or_deg)
  Demux/1 -> outer/1, [of_deg]
  Demux/3 -> outer1/1, [or_deg]
  Demux/2 -> inner1/1, [ir_deg]
  [if_deg] -> inner/1
  Mux/1 -> Out1/1
  Saturation1/1 -> [if_deg], Switch/2, YO equation/1(Steer)
  Speed/1 -> XO equation/1(In1)

== system SDV_HIL/Draft1/UDP Transmit PC -> VCU1/Subsystem/Torque Vectoring/Ca Calculations ==
  <Fz> : Inport
  1-D Lookup Table : Lookup_n-D  NumberOfTableDimensions=1  BreakpointsForDimension1=Breakpoints_Fz  Table=Cij  InternalRulePriority=Speed  RndMeth=Simplest
  Add : Sum
  Add1 : Sum
  Bus Creator2 : BusCreator  Inputs=2
  Demux : Demux
  Scope1 : Scope  Commented=on
      settings: ActiveDisplayYMinimum=151092.72809837208  ActiveDisplayYMaximum=177792.29609670336  DataLoggingVariableName=ScopeData_Cai
  Ca : Outport
  wires:
  Bus Creator2/1 -> Ca/1, Scope1/1  "Ca"
  Demux/1 -> Add/1  "FL"
  1-D Lookup Table/1 -> Demux/1
  Demux/2 -> Add/2  "FR"
  Demux/3 -> Add1/1  "RL"
  Add/1 -> Bus Creator2/1  "front"
  Demux/4 -> Add1/2  "RR"
  Add1/1 -> Bus Creator2/2  "rear"
  <Fz>/1 -> 1-D Lookup Table/1

== system SDV_HIL/Draft1/UDP Transmit PC -> VCU1/Subsystem/Torque Vectoring/Lower-Level Control ==
  Fx_total : Inport
  Mzd : Inport  Port=2
  delta_in : Inport  Port=3
  Fz : Inport  Port=4
  Constant : Constant  Value=4
  Constant1 : Constant  Value=mu
  Constant2 : Constant  Value=Tmax
  Display2 : Display  Commented=on
  Divide : Product  Inputs=*/
  Gain : Gain  Gain=R_eff
  Gain1 : Gain  Gain=4
  MATLAB Function1 : MATLAB Function  TreatAsAtomicUnit=on  SystemSampleTime=0.001
  Mux : Mux  Inputs=2
  Scope : Scope  Commented=on  NumInputPorts=2
      settings: ActiveDisplayYMinimum=-1280.000000001761  ActiveDisplayYMaximum=1280.0000000158495  DataLoggingVariableName=ScopeData44
  Scope1 : Scope  Commented=on  NumInputPorts=2
      settings: ActiveDisplayYMinimum=-9578.3971707250021  ActiveDisplayYMaximum=10211.837981002229  DataLoggingVariableName=ScopeData42
  Scope2 : Scope  Commented=on
      settings: ActiveDisplayYMinimum=-1.75  ActiveDisplayYMaximum=5.75  DataLoggingVariableName=ScopeData53
  Scope3 : Scope  Commented=on
      settings: ActiveDisplayYMinimum=-1  ActiveDisplayYMaximum=1  DataLoggingVariableName=ScopeData30
  Scope4 : Scope  Commented=on  NumInputPorts=3
      settings: ActiveDisplayYMinimum=-1734.1040462427745  ActiveDisplayYMaximum=1734.1040462427745  DataLoggingVariableName=ScopeData56
  Sum of Elements : Sum  Inputs=+
  Unit Delay : UnitDelay  InitialCondition=[0; 0; 0; 0]  SampleTime=-1  HasFrameUpgradeWarning=on
  TqMotorRef : Outport
  wires:
  Gain1/1 -> MATLAB Function1/5(Tshaft_max)
  Constant2/1 -> Gain1/1
  Mux/1 -> Scope3/1
  delta_in/1 -> MATLAB Function1/3(delta_in)
  Sum of Elements/1 -> Mux/2  "sum(Fx_opt)"
  Constant1/1 -> MATLAB Function1/6(mu)
  MATLAB Function1/3(Mx_total) -> Scope1/2  "Mx_total"
  Divide/1 -> TqMotorRef/1, Display2/1, Scope/2  "TqMotor"
  Constant/1 -> Divide/2
  MATLAB Function1/5(Fx_opt) -> Gain/1, Sum of Elements/1, Scope4/3, Unit Delay/1  "Fx_opt"
  Fz/1 -> MATLAB Function1/4(Fz)
  Mzd/1 -> Scope1/1, MATLAB Function1/2(Mzd)
  Fx_total/1 -> MATLAB Function1/1(Fx_total_ref), Mux/1
  Gain/1 -> Divide/1, Scope/1  "TqShaft"
  MATLAB Function1/4(exitflag) -> Scope2/1
  Unit Delay/1 -> MATLAB Function1/7(Fx_prev)
  MATLAB Function1/1(lb) -> Scope4/1  "lb"
  MATLAB Function1/2(ub) -> Scope4/2  "ub"

== system SDV_HIL/Draft1/UDP Transmit PC -> VCU1/Subsystem/Torque Vectoring/Reference Model ==
  delta_in : Inport
  Vx : Inport  Port=2
  Ca : Inport  Port=3
  Demux2 : Demux  Outputs=2
  Demux3 : Demux  Outputs=2
  Display : Display  Commented=on
  Draft : Subsystem  Commented=on
  Gain3 : Gain  Gain=-1
  Gain5 : Gain  Gain=-1
  Reference Model : MATLAB Function  TreatAsAtomicUnit=on
  Saturation Dynamic : simulink/Discontinuities/Saturation Dynamic  OutMin=[]  OutMax=[]  OutDataTypeStr=Inherit: Same as second input  OutDataType=fixdt(1, 16)  OutScaling=2^-10  DoSatur=off
  Saturation Dynamic1 : simulink/Discontinuities/Saturation Dynamic  OutMin=[]  OutMax=[]  OutDataTypeStr=Inherit: Same as second input  OutDataType=fixdt(1, 16)  OutScaling=2^-10  DoSatur=off
  Scope : Scope  Commented=on
      settings: ActiveDisplayYMinimum=-0.010237730942831622  ActiveDisplayYMaximum=0.0448211063407787  DataLoggingVariableName=ScopeData35
  Scope1 : Scope  Commented=on  NumInputPorts=2
      settings: ActiveDisplayYMinimum=-0.010237730942831622  ActiveDisplayYMaximum=0.0448211063407787  DataLoggingVariableName=ScopeData43
  Scope2 : Scope  Commented=on  NumInputPorts=2
      settings: ActiveDisplayYMinimum=-1  ActiveDisplayYMaximum=1  DataLoggingVariableName=ScopeData45
  Scope3 : Scope  Commented=on  NumInputPorts=2
      settings: ActiveDisplayYMinimum=-0.28358581685431428  ActiveDisplayYMaximum=0.28405537038366757  DataLoggingVariableName=ScopeData41
  Selector : Selector  InputPortWidth=2  IndexOptions=Index vector (dialog)  Indices=[1]  OutputSizes=1
  r&beta Limiter : Subsystem
  r_des : Outport
  beta_des : Outport  Port=2
  wires:
  Demux3/1 -> Scope1/1, Saturation Dynamic/2  "r_des"
  Demux2/1 -> Reference Model/3(Caf)
  Demux2/2 -> Reference Model/4(Car)
  Vx/1 -> r&beta Limiter/1(Vx), Reference Model/2(Vx)
  Demux3/2 -> Scope2/1, Saturation Dynamic1/2  "beta_des"
  delta_in/1 -> Selector/1
  Ca/1 -> Demux2/1
  Reference Model/1(y) -> Scope/1, Demux3/1  "r & beta_des"
  Gain3/1 -> Saturation Dynamic/3
  Saturation Dynamic/1 -> Display/1, r_des/1, Scope3/1, Scope1/2  "r_desUnsat"
  Gain5/1 -> Saturation Dynamic1/3
  Saturation Dynamic1/1 -> Scope2/2, beta_des/1, Scope3/2  "beta_desUnsat"
  r&beta Limiter/1(rLim) -> Gain3/1, Saturation Dynamic/1
  r&beta Limiter/2(betaLim) -> Saturation Dynamic1/1, Gain5/1
  Selector/1 -> Reference Model/1(delta_in)
